simulink model "CRC_chain"  (R2025b)
settings: Solver=VariableStepAuto  StartTime=0.0  StopTime=inf  RelTol=1e-3
libraries: simulink x4, hdlsllib x3, commhdlcrc x2, commseqgen3 x1
settings Model: PacingRate=10  Creator=strog  LastModifiedBy=strog
settings OptimizationCC: BlockReduction=off  ConditionallyExecuteInputs=off

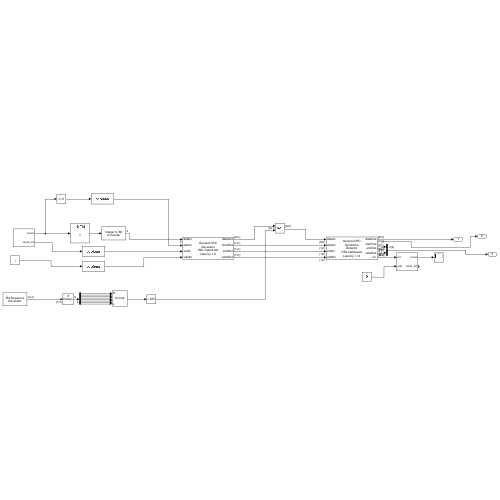
[thumbnail: Simulink's stored preview of the top-level diagram]
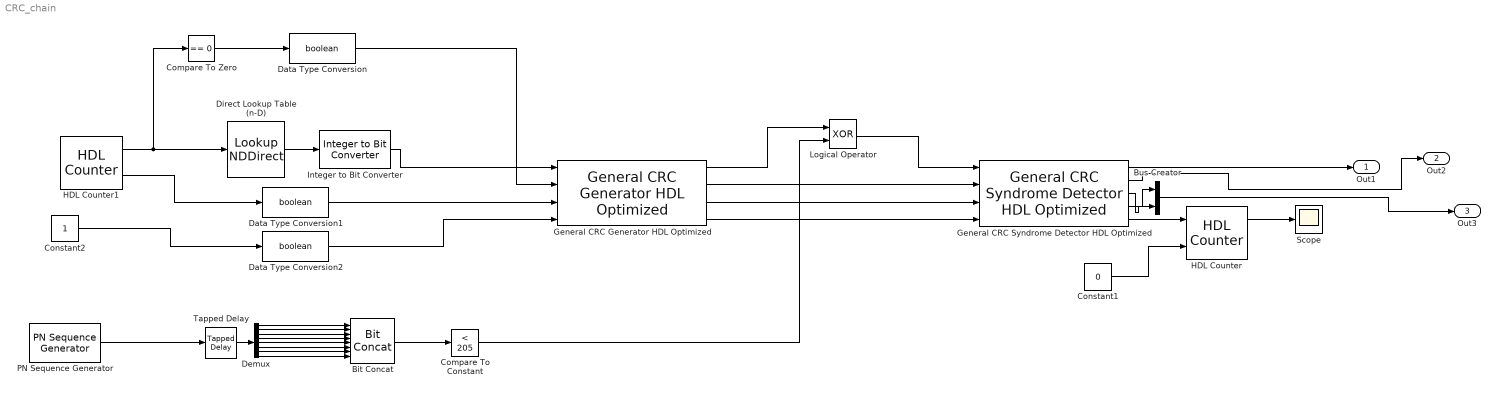
== system CRC_chain ==
  Bit Concat : hdlsllib/Logic and Bit Operations/Bit Concat  numInputs=8
  Bus Creator : BusCreator  Inputs=2
  Compare To Constant : simulink/Logic and Bit Operations/Compare To Constant  relop=<  const=205  OutDataTypeStr=boolean
  Compare To Zero : simulink/Logic and Bit Operations/Compare To Zero  relop===  OutDataTypeStr=boolean
  Constant1 : Constant  Value=0  OutDataTypeStr=boolean
  Constant2 : Constant  OutDataTypeStr=boolean
  Data Type Conversion : DataTypeConversion  OutDataTypeStr=boolean  SaturateOnIntegerOverflow=off  RndMeth=Floor
  Data Type Conversion1 : DataTypeConversion  OutDataTypeStr=boolean  SaturateOnIntegerOverflow=off  RndMeth=Floor
  Data Type Conversion2 : DataTypeConversion  OutDataTypeStr=boolean  SaturateOnIntegerOverflow=off  RndMeth=Floor
  Demux : Demux  Outputs=8
  Direct Lookup Table (n-D) : LookupNDDirect  NumberOfTableDimensions=1  Table=[72, 101, 108, 108, 111]  TableDataTypeStr=uint8
  General CRC Generator HDL Optimized : commhdlcrc/General CRC Generator HDL Optimized  Polynomial=polyCoeffs  InitialState=1  DirectMethod=on  ReflectInput=on  ReflectCRCChecksum=on  FinalXORValue=ones(1, 32)  SimulateUsing=Code generation
  General CRC Syndrome Detector HDL Optimized : commhdlcrc/General CRC Syndrome Detector HDL Optimized  Polynomial=polyCoeffs  InitialState=1  DirectMethod=on  ReflectInput=on  ReflectCRCChecksum=on  FinalXORValue=ones(1, 32)  SimulateUsing=Code generation
  HDL Counter : hdlsllib/Sources/HDL Counter  CountType=Count limited  CountInit=0  CountStep=1  CountMax=25  CountFromType=Initial value  CountFrom=0  CountResetPort=on  CountLoadPort=off  CountEnbPort=on  CountDirPort=off  CountHitOutputPort=on  CountDataType=Unsigned  CountWordLen=8  CountFracLen=0  CountSampTime=uint8(1)
  HDL Counter1 : hdlsllib/Sources/HDL Counter  CountType=Count limited  CountInit=0  CountStep=1  CountMax=4  CountFromType=Initial value  CountFrom=0  CountResetPort=off  CountLoadPort=off  CountEnbPort=off  CountDirPort=off  CountHitOutputPort=on  CountDataType=Unsigned  CountWordLen=8  CountFracLen=0  CountSampTime=1
  Integer to Bit Converter : simulink/Logic and Bit Operations/Integer to Bit Converter  nbits=8  signedInputValues=Unsigned  bitOrder=MSB first  outDtype=boolean
      settings: LibrarySourceBlock=|
      | commutil2/Integer to Bit
      | Converter
  Logical Operator : Logic  Operator=XOR  AllPortsSameDT=off  OutDataTypeStr=boolean
  PN Sequence Generator : commseqgen3/PN Sequence Generator  poly='z^6 + z + 1'  ini_sta=[0 0 0 0 0 1]  outBitMaskSource=Dialog parameter  shift=0  outVarSiz=off  maxOutSizeMode=Dialog parameter  maxOutSize=[10 1]  Ts=1  sampPerFrame=1  reset=off  bitPackedOutputs=off  outDataType=boolean  numPackedBits=8  bitPackDataSigned=off  bitPackedOutDType=double
      settings: LibrarySourceBlock=|
      | commhdlsource/PN Sequence
      | Generator
  Scope : Scope
      settings: ActiveDisplayYMinimum=-1  ActiveDisplayYMaximum=1  DataLoggingVariableName=ScopeData2  DataLoggingSaveFormat=Array
  Tapped Delay : simulink/Discrete/Tapped Delay  vinit=0.0  samptime=-1  NumDelays=8  DelayOrder=Oldest  includeCurrent=off
  Out1 : Outport
  Out2 : Outport  Port=2
  Out3 : Outport  Port=3
  wires:
  Constant1/1 -> HDL Counter/2
  General CRC Syndrome Detector HDL Optimized/4 -> Bus Creator/1
  General CRC Syndrome Detector HDL Optimized/3 -> Bus Creator/2
  General CRC Generator HDL Optimized/1 -> Logical Operator/1
  Logical Operator/1 -> General CRC Syndrome Detector HDL Optimized/1
  General CRC Generator HDL Optimized/2 -> General CRC Syndrome Detector HDL Optimized/2
  General CRC Generator HDL Optimized/4 -> General CRC Syndrome Detector HDL Optimized/4
  General CRC Syndrome Detector HDL Optimized/5 -> HDL Counter/1
  General CRC Generator HDL Optimized/3 -> General CRC Syndrome Detector HDL Optimized/3
  HDL Counter/1 -> Scope/1
  Compare To Constant/1 -> Logical Operator/2
  HDL Counter1/1 -> Compare To Zero/1, Direct Lookup Table (n-D)/1
  Direct Lookup Table (n-D)/1 -> Integer to Bit Converter/1
  HDL Counter1/2 -> Data Type Conversion1/1
  Constant2/1 -> Data Type Conversion2/1
  Compare To Zero/1 -> Data Type Conversion/1
  PN Sequence Generator/1 -> Tapped Delay/1
  Bit Concat/1 -> Compare To Constant/1
  Tapped Delay/1 -> Demux/1
  Demux/1 -> Bit Concat/1
  Demux/2 -> Bit Concat/2
  Demux/3 -> Bit Concat/3
  Demux/4 -> Bit Concat/4
  Demux/5 -> Bit Concat/5
  Demux/6 -> Bit Concat/6
  Demux/7 -> Bit Concat/7
  Demux/8 -> Bit Concat/8
  Data Type Conversion/1 -> General CRC Generator HDL Optimized/2
  Data Type Conversion1/1 -> General CRC Generator HDL Optimized/3
  Data Type Conversion2/1 -> General CRC Generator HDL Optimized/4
  Integer to Bit Converter/1 -> General CRC Generator HDL Optimized/1
  General CRC Syndrome Detector HDL Optimized/1 -> Out1/1
  General CRC Syndrome Detector HDL Optimized/2 -> Out2/1
  Bus Creator/1 -> Out3/1
